simulink model "pff"  (Simulink 8.1)
settings: Solver=ode45  StartTime=0.0  StopTime=10.0  RelTol=1e-3
settings Model: Creator=Mihail  LastModifiedBy=Mihail
settings DebuggingCC: FcnCallInpInsideContextMsg=EnableAllAsWarning
settings GRTTargetCC: CombineOutputUpdateFcns=on  GRTInterface=off

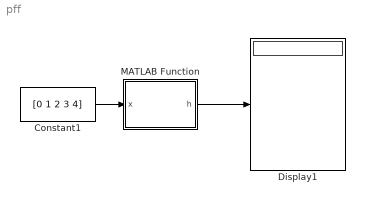
== system pff ==
  Constant1 : Constant  Value=[0 1 2 3 4]
  Display1 : Display
  MATLAB Function : MATLAB Function  TreatAsAtomicUnit=on
  wires:
  MATLAB Function/1(h) -> Display1/1
  Constant1/1 -> MATLAB Function/1(x)

== matlab function MATLAB Function ==
  data: x input double; h output double
function h = fcn(x)
%#codegen

h=x;
